simulink model "house2"  (R2022b)
settings: Solver=VariableStepAuto  StartTime=0.0  StopTime=60  RelTol=1e-3
libraries: vrlib x1
settings Model: Creator=Abdiladif Hassan  LastModifiedBy=Administrator
settings OptimizationCC: ReuseModelBlockBuffer=on

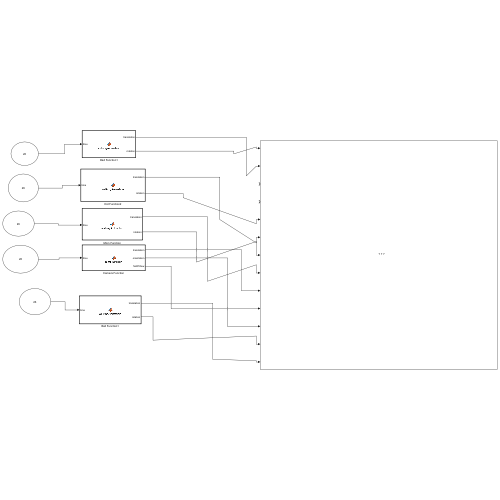
[thumbnail: Simulink's stored preview of the top-level diagram]
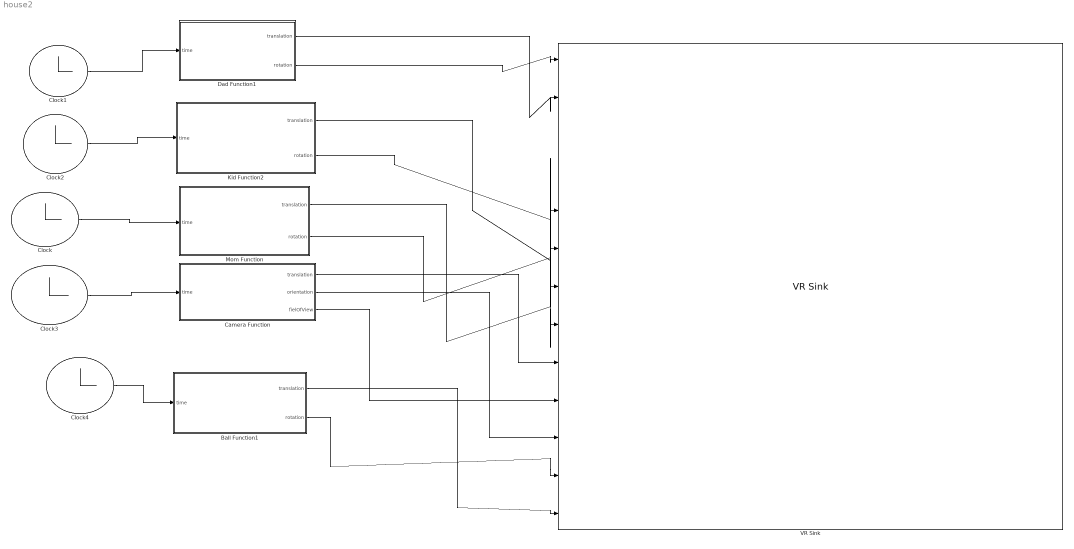
== system house2 ==
  Ball Function1 : MATLAB Function  TreatAsAtomicUnit=on
  Camera Function : MATLAB Function  TreatAsAtomicUnit=on
  Clock{,1..4} (5 alike) : Clock
  Dad Function1 : MATLAB Function  TreatAsAtomicUnit=on
  Kid Function2 : MATLAB Function  TreatAsAtomicUnit=on
  Mom Function : MATLAB Function  TreatAsAtomicUnit=on
  VR Sink : vrlib/VR Sink  InstantiateOnLoad=on  SampleTime=0.1  ViewEnable=on  RemoteChange=off  RemoteView=off  FieldsWritten=dad_TRANSFORM.rotation.4.1.1.double#dad_TRANSFORM.translation.3.1.1.double#window_012_TRANSFORM.rotation.4.1.1.double#window_012_TRANSFORM.translation.3.1.1.double#kid1_TRANSFORM.rotation.4.1.1.double#kid1_TRANSFORM.translation.3.1.1.double#mom_TRANSFORM.rotation.4.1.1.double#mom_TRANSFORM.translation.3.1.1.double#Camera_TRANSFORM.translation.3.1.1.double#CA_Camera.fieldOfView.1.1.1.double#CA_Camera.orientation.4.1.1.double#ball_TRANSFORM.rotation.4.1.1.double#ball_TRANSFORM.translation.3.1.1.double  WorldFileName=house31.x3d  AutoView=on  VideoDimensions=[]  AllowVariableSize=off  FigureProperties="{'Position', 'Name', 'Viewpoint', 'CameraBound', 'CameraDirection', 'CameraPosition', 'CameraUpVector', 'ZoomFactor', 'Antialiasing', 'Headlight', 'Lighting', 'NavPanel', 'Sound', 'StatusBar', 'Stereo3D', 'Stereo3DCameraOffset', 'Stereo3DHIT', 'ToolBar', 'Textures', 'Transparency', 'Triad', 'Wireframe', 'NavZones', 'NavMode', 'NavSpeed', 'CaptureFileFormat', 'CaptureFileName', 'Record2DCompressMethod', 'Record2DCompressQuality', 'Record2D', 'Record2DFileName', 'Record2DFPS'; [1.0000000000000000e+00   7.6000000000000000e+01   1.3660000000000000e+03   5.9300000000000000e+02], '', '_untitled_1', 'on', [-5.3062668424327386e-02   3.5477019908180918e-02  -9.9796078794616183e-01], [3.8843203743748589e-01  -8.5055065276027619e-01   4.6981484530767133e+01], [2.5098512747740520e-03   9.9937029592031612e-01   3.5393675688114551e-02], [1.2100000000000002e+00], 'off', 'on', 'on', 'halfbar', 'on', 'on', 'off', [1.0000000149011612e-01], [0.0000000000000000e+00], 'on', 'on', 'on', 'none', 'off', 'off', 'fly', 'normal', 'tif', '%f_anim_%n.tif', 'auto', [7.5000000000000000e+01], 'off', '%f_anim_%n.avi', 'auto'}"
  wires:
  Clock/1 -> Mom Function/1(time)
  Clock1/1 -> Dad Function1/1(time)
  Clock2/1 -> Kid Function2/1(time)
  Clock3/1 -> Camera Function/1(time)
  Clock4/1 -> Ball Function1/1(time)
  Dad Function1/2(rotation) -> VR Sink/1
  Dad Function1/1(translation) -> VR Sink/2
  Kid Function2/2(rotation) -> VR Sink/5
  Kid Function2/1(translation) -> VR Sink/6
  Mom Function/2(rotation) -> VR Sink/7
  Mom Function/1(translation) -> VR Sink/8
  Camera Function/1(translation) -> VR Sink/9
  Camera Function/2(orientation) -> VR Sink/11
  Ball Function1/2(rotation) -> VR Sink/12
  Ball Function1/1(translation) -> VR Sink/13
  Camera Function/3(fielOfView) -> VR Sink/10

== matlab function house2/Dad Function1 ==
  data: time input; translation output; rotation output
function [translation, rotation] = walkingAnimation(time)
    % Initial position
    initial_translation = [-2.9294, 0.054634, -9.637];
    initial_rotation = [-0.31548, 0.63089, 0.70884, 2.5312];
    
    % Adjust the walking animation parameters based on your requirements
    
    
    % Initialize translation and rotation values
    translation = initial_translation;
    rotation = initial_rotation;
    
    % Check if time is within the walking duration (10 seconds)
    if time <= 6
        % Update the x-coordinate of the translation for straight walking
        translation(1) = initial_translation(1) + 0.8 * time; % Adjust the factor (0.1) as needed for speed
        
        % Set rotation to keep the character upright (no turning)
        rotation = initial_rotation;
    else
        % Stop walking after 10 seconds by keeping the translation constant
       translation(1) = initial_translation(1) + 0.9 * 6; % Adjust the final position as needed
       rotation = initial_rotation;
    end
end

== matlab function house2/Mom Function ==
  data: time input; translation output; rotation output
function [translation, rotation] = walkingAnimation(time)
    % Initial position
    initial_translation = [-3.2584, 0.13427, -7.8401];
    initial_rotation = [-0.64928, 0.57913, 0.493, 2.0828];
    
    % Adjust the walking animation parameters based on your requirements
    %walking_angle = sin(2*pi*time/10); % Modify this based on your walking animation
    
    % Initialize translation and rotation values
    translation = initial_translation;
    rotation = initial_rotation;

    % Calculate rotated quaternion
    q0 = initial_rotation(1);
    q1 = initial_rotation(2);
    q2 = initial_rotation(3);
    q3 = initial_rotation(4);
    
    rotated_q0 = q0 * sin(pi/4);
    rotated_q1 = q0 * sin(pi/4);
    rotated_q2 = q0 * sin(pi/4);
    rotated_q3 = q3;
    
    rotated_rotation = [rotated_q0, rotated_q1, rotated_q2, rotated_q3];

    % Check if time is within the walking duration
    if time <= 8
        % Update translation for straight walking
        translation(1) = translation(1) + 1 * time; % Adjust the factor (0.1) as needed for speed
    elseif time > 8 && time <= 17
        % Rotate and continue straight walking
        translation(1) = translation(1) + 8;
        rotation = rotated_rotation;
    elseif time > 17 && time <= 21
        % Rotate and move diagonally with a loop
        rotation = [-0.64928, 0.57913, 0.493, 2.0828];
        translation(1) = translation(1) + 8;
        translation(2) = translation(2) + 0.25;
       
       
        translation(3) = translation(3) + 1.5*(time-17); % Adjust the factor (0.1) as needed for speed
            
        
    elseif time > 21 && time <= 30
        % Rotate and move diagonally
        rotation = rotated_rotation;
        translation(1) = translation(1) + 8;
        translation(2) = translation(2) + 0.25;
      
        translation(3) = translation(3) + 1.5 * 4;
        translation = [translation(1)-1, translation(2), translation(3)];
        %translation(1) = initial_translation(1) + 0.5 * (time-21);
    end
end

== matlab function house2/Kid Function2 ==
  data: time input; translation output; rotation output
function [translation, rotation] = walkingAnimation(time)
    % Initial position
    initial_translation = [-3.20238, 0.082384, -11.6038];
    initial_rotation = [-0.60466, 0.5304, 0.59419,1.879];
    
    % Adjust the walking animation parameters based on your requirements
    
    % Slow down the animation (increase the denominator for slower motion)
    walking_angle = sin(2*pi*time/10); % Modify this based on your walking animation
    
    % Initialize translation and rotation values
    translation = initial_translation;
    rotation = initial_rotation;
    
    % Check if time is within the walking duration (10 seconds)
    if time <= 5
        % Update the x-coordinate of the translation for straight walking
        translation(1) = initial_translation(1) + 0.7 * time; % Adjust the factor (0.1) as needed for speed
        
        % Set rotation to keep the character upright (no turning)
        rotation = initial_rotation;
    else
        % Stop walking after 10 seconds by keeping the translation constant
        translation(1) = initial_translation(1) + 0.9 * 5; % Adjust the final position as needed
        rotation = initial_rotation;
    end
end

== matlab function house2/Camera Function ==
  data: time input; translation output; orientation output; fielOfView output
function [translation, orientation, fielOfView] = cameraMotion(time)
    % Initial position
    initial_translation = [16.907, 19.1728, -68.6527];
    initial_orientation = [-0.43, -0.89, 0.14, 0];
    initial_fielOfView = 0.443;

    % Adjust the walking animation parameters based on your requirements
    
    % Initialize translation and rotation values
    translation = initial_translation;
    orientation = initial_orientation;
    fielOfView = initial_fielOfView;


    % Check if time is within the walking duration (25 seconds)
    if time <= 10
        % Update the x-coordinate of the translation for straight walking
       % translation(3) = initial_translation(3) + 5 * 10; % Adjust the factor (0.1) as needed for speed
       % translation(2) = initial_translation(2) - 10;
       % translation(1) = initial_translation(1) - 12;
        translation = [4.907, 9.1728, -18.6527];
        orientation = [-0.43, -0.89, 0.14, 1];
    elseif time > 10 && time <= 15
        % Continue straight walking animation
        %translation(3) = initial_translation(3) + 4 * time;
        %translation(2) = initial_translation(2) - 17;
        %translation(1) = initial_translation(1) - 12;
        translation = [4.907, 2.1728, -8.6527];
        orientation = [-0.43, -0.89, 0.14, 1];
    elseif time > 15 && time <= 22
        % Continue straight walking animation with updated orientation
        %translation(3) = initial_translation(3) + 3.5 * time;
        %translation(2) = initial_translation(2) - 25.1728;
        %translation(1) = initial_translation(1) + 5;
        translation = [-2.307, -6, 27.3475];

        orientation = [-0.43, -0.89, 0.14, 0];
        fielOfView = 0.123;
    elseif time >22 && time <=30
        %translation(3) = initial_translation(3) + 3.5 * time;
        %translation(2) = initial_translation(2) - 25.1728;
        %translation(1) = initial_translation(1) - time;
         translation = [-6.307, -7.4, 28.3475];
         translation(3) = translation(3) + 12.2;
        orientation = [-0.43, -0.89, 0.14, 0];
        fielOfView = 0.43;

    end
end

== matlab function house2/Ball Function1 ==
  data: time input; translation output; rotation output
function [translation, rotation] = walkingAnimation(time)
    % Initial position
    initial_translation = [-3.20238, 0.082384, -11.6038];
    initial_rotation = [-0.60466, 0.5304, 0.59419,1.879];
    
    % Adjust the walking animation parameters based on your requirements
    
    % Slow down the animation (increase the denominator for slower motion)
    walking_angle = sin(2*pi*time/10); % Modify this based on your walking animation
    
    % Initialize translation and rotation values
    translation = initial_translation;
     translation(2) = initial_translation(2) + 10;
    rotation = initial_rotation;
    
    % Check if time is within the walking duration (10 seconds)
    if time <= 10
        % Update the x-coordinate of the translation for straight walking
        %translation(1) = initial_translation(1) + 0.9 * time; % Adjust the factor (0.1) as needed for speed
        
        % Set rotation to keep the character upright (no turning)
        translation(1) = initial_translation(1) + 0.9 * 10;
        rotation = initial_rotation;
    else
        % Stop walking after 10 seconds by keeping the translation constant
        translation(1) = initial_translation(1) + 0.9 * 10; % Adjust the final position as needed
        rotation = initial_rotation;
    end
end
